simulink subsystem "CalculateNormalCriticalRBV"  (R2023a)
settings: Solver=VariableStepAuto  StartTime=0.0  StopTime=10.0  RelTol=1e-3
libraries: SignalEditorBlockLib x1
settings Model: Creator=ppatel  LastModifiedBy=ppatel

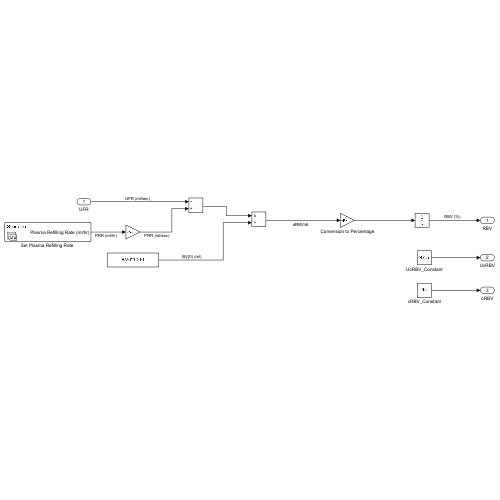
[thumbnail: Simulink's stored preview of the top-level diagram]
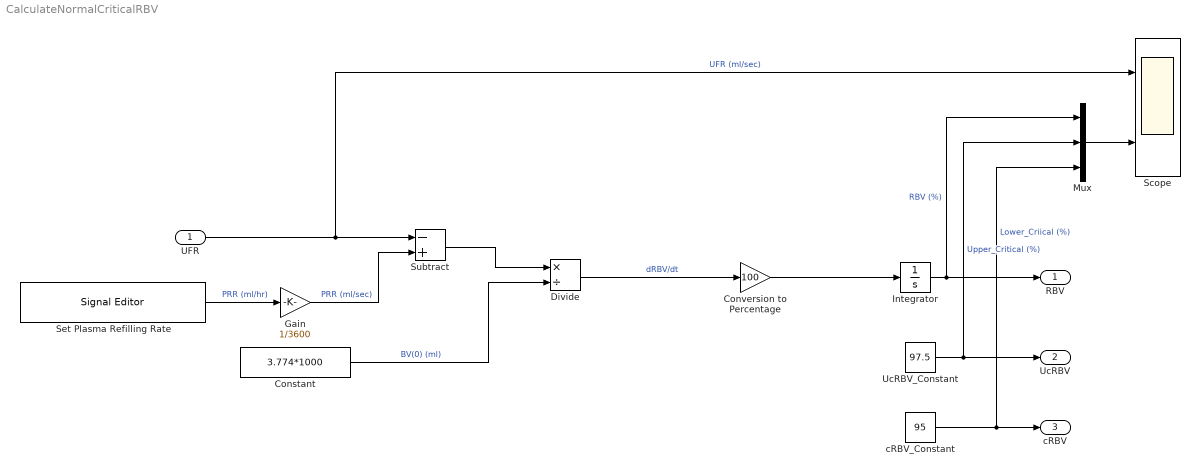
== system CalculateNormalCriticalRBV ==
  UFR : Inport
  Constant : Constant  Value=3.774*1000
  Conversion to Percentage : Gain  Gain=100
  Divide : Product  Inputs=*/
  Gain : Gain  Gain=1/3600
  Integrator : Integrator  InitialCondition=100
  Mux : Mux  Inputs=3
  Scope : Scope  NumInputPorts=2
  "Set Plasma Refilling Rate " : SignalEditorBlockLib/Signal Editor  FileName=dialysisDemo_PRR.mat  ActiveScenario=Scenario  ActiveSignal=Plasma Refilling Rate (ml/hr)  IsBus=off  OutputBusObjectStr=Bus: BusObject  SampleTime=0  Interpolate=off  ZeroCross=off  OutputAfterFinalValue=Setting to zero  Unit=inherit  PreserveSignalName=on  ApplySigPropsToAllScenarios=on
  Subtract : Sum  Inputs=-+
  UcRBV_Constant : Constant  Value=97.5
  cRBV_Constant : Constant  Value=95
  RBV : Outport
  UcRBV : Outport  Port=2
  cRBV : Outport  Port=3
  wires:
  Conversion to Percentage/1 -> Integrator/1
  "Set Plasma Refilling Rate "/1 -> Gain/1  "PRR (ml/hr)"
  Subtract/1 -> Divide/1
  Gain/1 -> Subtract/2  "PRR (ml/sec)"
  Divide/1 -> Conversion to Percentage/1  "dRBV/dt"
  Constant/1 -> Divide/2  "BV(0) (ml)"
  UFR/1 -> Subtract/1, Scope/1  "UFR (ml/sec)"
  Integrator/1 -> RBV/1, Mux/1  "RBV (%)"
  UcRBV_Constant/1 -> UcRBV/1, Mux/2  "Upper_Critical (%)"
  cRBV_Constant/1 -> cRBV/1, Mux/3  "Lower_Criical (%)"
  Mux/1 -> Scope/2
